simulink model "part_d_nonlinear"  (R2024b)
settings: Solver=VariableStepAuto  StartTime=0.0  StopTime=1000  RelTol=1e-3
values from neighbouring files (symbols this model uses):
  g = sym("g")    [part_E.m]    (also in part_F.m = 9.8; part_G.m = 9.8; part_b.m; part_c.m)
  l1 = sym("l1")    [part_E.m]    (also in part_F.m = 20; part_G.m = 20; part_b.m; part_c.m)
  l2 = sym("l2")    [part_E.m]    (also in part_F.m = 10; part_G.m = 10; part_b.m; part_c.m)
  M = sym("M")    [part_E.m]    (also in part_F.m = 1000; part_G.m = 1000; part_b.m; part_c.m)
  m1 = sym("m1")    [part_E.m]    (also in part_F.m = 100; part_G.m = 100; part_b.m; part_c.m)
  m2 = sym("m2")    [part_E.m]    (also in part_F.m = 100; part_G.m = 100; part_b.m; part_c.m)
undefined symbols (not defined in the file or in its folder): K
settings Model: Creator=timsweeney  LastModifiedBy=timsweeney

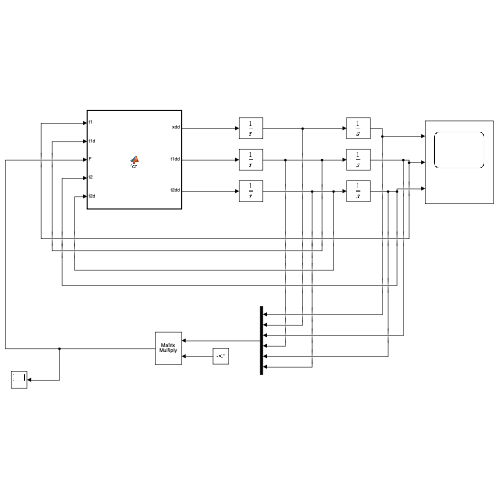
[thumbnail: Simulink's stored preview of the top-level diagram]
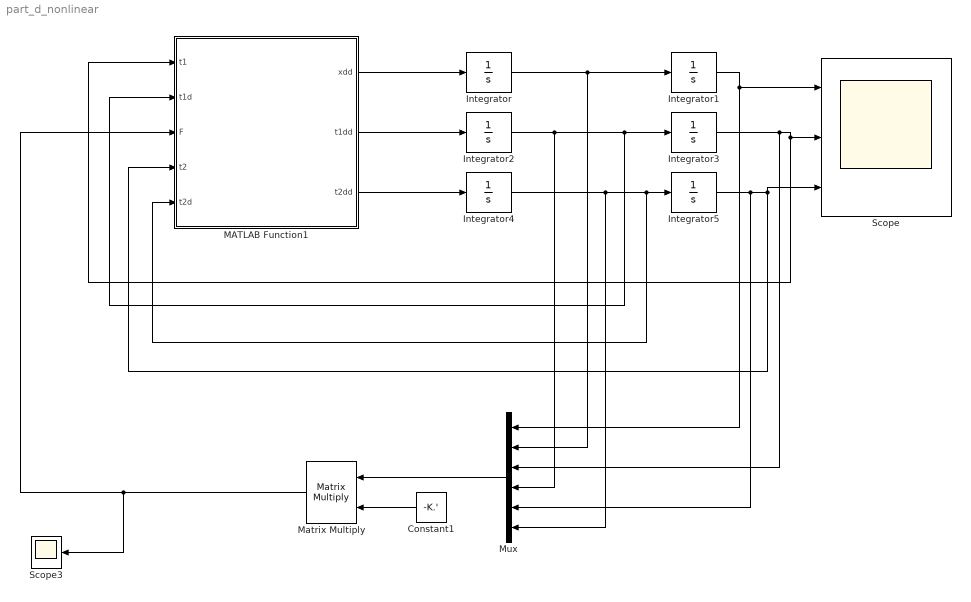
== system part_d_nonlinear ==
  Constant1 : Constant  Value=-K.'
  Integrator{,1..2,4} (4 alike) : Integrator
  Integrator3 : Integrator  InitialCondition=pi/10
  Integrator5 : Integrator  InitialCondition=-pi/10
  MATLAB Function1 : MATLAB Function  TreatAsAtomicUnit=on
  Matrix Multiply : Product  Multiplication=Matrix(*)
  Mux : Mux  Inputs=6
  Scope : Scope  NumInputPorts=3
  Scope3 : Scope
  wires:
  MATLAB Function1/1(xdd) -> Integrator/1
  MATLAB Function1/2(t1dd) -> Integrator2/1
  Integrator/1 -> Mux/2, Integrator1/1
  Integrator2/1 -> Mux/4, MATLAB Function1/2(t1d), Integrator3/1
  Integrator4/1 -> Mux/6, MATLAB Function1/5(t2d), Integrator5/1
  Integrator1/1 -> Mux/1, Scope/1
  Integrator3/1 -> Mux/3, Scope/2, MATLAB Function1/1(t1)
  Integrator5/1 -> Mux/5, Scope/3, MATLAB Function1/4(t2)
  Matrix Multiply/1 -> Scope3/1, MATLAB Function1/3(F)
  MATLAB Function1/3(t2dd) -> Integrator4/1
  Mux/1 -> Matrix Multiply/1
  Constant1/1 -> Matrix Multiply/2

== matlab function part_d_nonlinear/MATLAB Function1 ==
  data: t1 input; t1d input; F input; t2 input; t2d input; xdd output; t1dd output; m1 parameter; m2 parameter; l1 parameter; l2 parameter; M parameter; g parameter; t2dd output
function [xdd, t1dd, t2dd] = fcn( t1, t1d, F, t2, t2d, m1, m2, l1, l2, M, g)

xdd = (F - m1*l1*sin(t1)*t1d^2 - m2*l2*sin(t2)*t2d^2 - m1*g*cos(t1)*sin(t1) - m2*g*cos(t2)*sin(t2)) ...
       / ...
      (M + m1*sin(t1)^2 + m2*sin(t2)^2);
t1dd = (1/l1) * (cos(t1)*xdd - g*sin(t1));
t2dd = (1/l2) * (cos(t2)*xdd - g*sin(t2));

% t2dd = 0;
